simulink model "EX_display_1"  (Simulink 4.00)
settings: Solver=ode45  StartTime=0.0  StopTime=10  MaxStep=0.01  RelTol=1e-3
settings Model: LastModifiedBy=Администратор

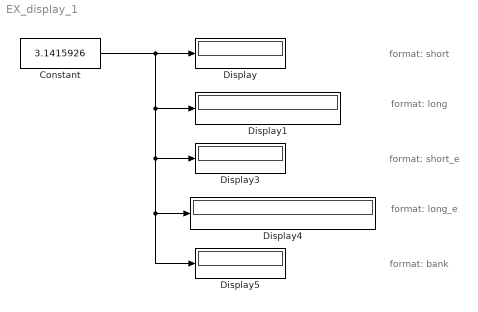
== system EX_display_1 ==
  note: format: short
  note: format: long
  note: format: short_e
  note: format: long_e
  note: format: bank
  Constant : Constant  Value=3.1415926
  Display{,1,3..5} (5 alike) : Display
      Display settings: Format=short
      Display3 settings: Format=short_e
      Display4 settings: Format=long_e
      Display5 settings: Format=bank
  wires:
  Constant/1 -> Display/1, Display1/1, Display3/1, Display4/1, Display5/1
